simulink model "esp32_udp_testsend"  (R2024b)
settings: Solver=FixedStepDiscrete  StartTime=0.0  StopTime=0.02  FixedStep=0.01  RelTol=1e-3
libraries: dspnetwork x1
settings Model: Creator=Anny  LastModifiedBy=Anny

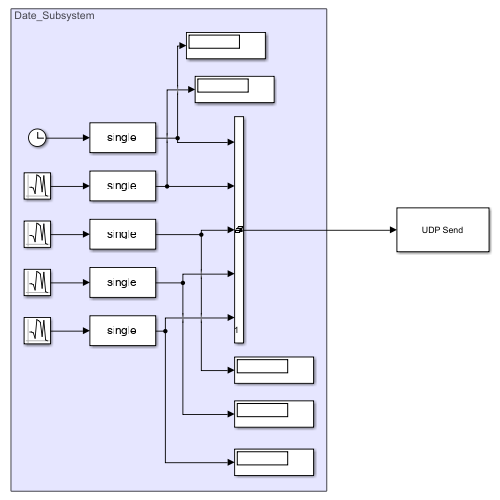
[thumbnail: Simulink's stored preview of the top-level diagram]
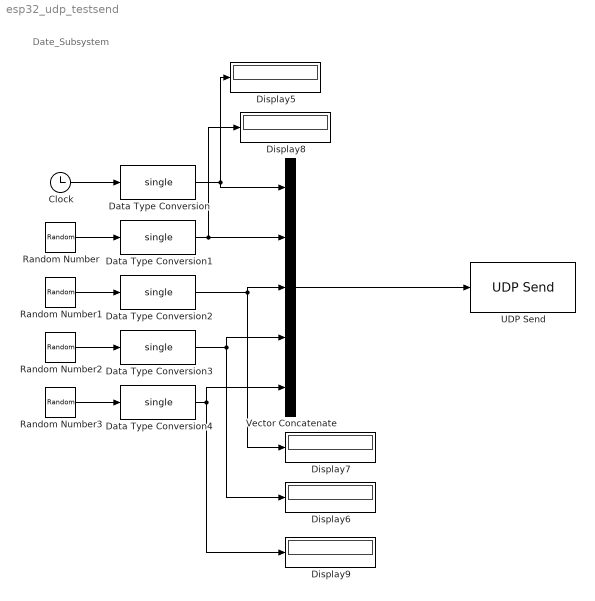
== system esp32_udp_testsend ==
  note: Date_Subsystem
  Clock : Clock
  Data Type Conversion{,1..4} (5 alike) : DataTypeConversion  OutDataTypeStr=single  SaturateOnIntegerOverflow=off  RndMeth=Floor
  Display{5..9} (5 alike) : Display
  Random Number : RandomNumber  Seed=1  SampleTime=0.01
  Random Number1 : RandomNumber  Seed=5  SampleTime=.01
  Random Number2 : RandomNumber  Seed=8  SampleTime=0.01
  Random Number3 : RandomNumber  Seed=11  SampleTime=0.01
  UDP Send : dspnetwork/UDP Send  remoteURL='172.20.10.2'  remotePort=12345  localURL='0.0.0.0'  localPortSource=Specify via dialog  localPort=25001  sendBufferSize=1024  sampletime=-1  blockPlatform=[]  separateLengthPort=0
      settings: LibrarySourceBlock=dspsnks4/UDP Send
  Vector Concatenate : Concatenate  NumInputs=5  Mode=Multidimensional array
  wires:
  Data Type Conversion4/1 -> Vector Concatenate/5, Display9/1
  Data Type Conversion2/1 -> Vector Concatenate/3, Display7/1
  Random Number1/1 -> Data Type Conversion2/1
  Clock/1 -> Data Type Conversion/1
  Data Type Conversion1/1 -> Vector Concatenate/2, Display8/1
  Data Type Conversion3/1 -> Vector Concatenate/4, Display6/1
  Random Number3/1 -> Data Type Conversion4/1
  Random Number2/1 -> Data Type Conversion3/1
  Data Type Conversion/1 -> Vector Concatenate/1, Display5/1
  Random Number/1 -> Data Type Conversion1/1
  Vector Concatenate/1 -> UDP Send/1
